simulink model "C_3_2020b"  (R2021a)
settings: Solver=VariableStepAuto  StartTime=0.0  StopTime=10.0  RelTol=1e-3
undefined symbols (not defined in the file or in its folder): pendubot_eqt, pendubot_reg, Ts
libraries: simulink x2
settings Model: Creator=afons  LastModifiedBy=Colin
settings SolverCC: AlgebraicLoopSolver=TrustRegion
settings DebuggingCC: UnconnectedInputMsg=none  UnconnectedOutputMsg=none  UnconnectedLineMsg=none  SFMachineParentedDataDiag=warning
settings ModelReferenceCC: EnableRefExpFcnMdlSchedulingChecks=off
settings RTWCC: Description=Generic Real-Time Target

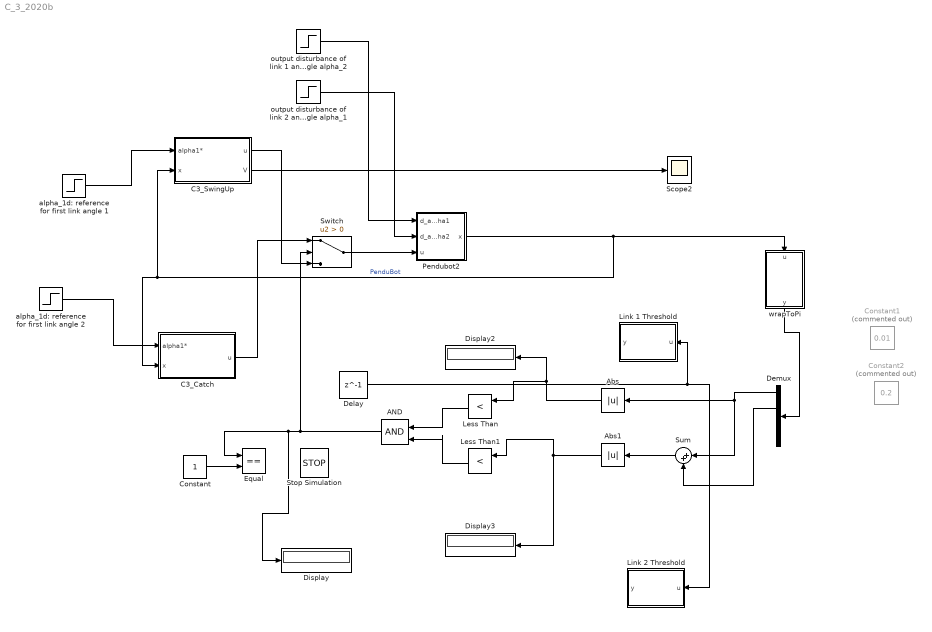
== system C_3_2020b ==
  AND : Logic  IconShape=distinctive  AllPortsSameDT=off  OutDataTypeStr=boolean
  Abs : Abs
  Abs1 : Abs
  C3_Catch : Subsystem
  C3_SwingUp : Subsystem
  Constant : Constant
  Constant1 : Constant  Commented=on  Value=0.01
  Constant2 : Constant  Commented=on  Value=0.2
  Delay : Delay  DelayLength=1
  Demux : Demux
  Display : Display
  Display2 : Display
  Display3 : Display
  Equal : RelationalOperator  Operator===  OutDataTypeStr=boolean  RndMeth=Simplest
  Less Than : RelationalOperator  Operator=<  OutDataTypeStr=boolean  RndMeth=Simplest
  Less Than1 : RelationalOperator  Operator=<  OutDataTypeStr=boolean  RndMeth=Simplest
  Link 1 Threshold : MATLAB Function  TreatAsAtomicUnit=on
  Link 2 Threshold : MATLAB Function  TreatAsAtomicUnit=on
  Pendubot2 : Subsystem  mask(Pendubot){x10=0, x20=0, x30=0, x40=0, Ts=Ts}
      mask prompts: x10 "Initial angle of link 1:"; x20 "Initial angular speed for link 1 :"; x30 "Initial angle of link 2 :"; x40 "Initial angular speed for link 2 :"; Ts "Sampling time [s] :"
      mask help: Initial conditions (initial state)
      mask Display:
      | plot(0.1*[1 9],0.1*[1 1])
      | plot(0.1*[1.5 1.5 8.5 8.5],0.1*[1 4 4 1])
      | plot(0.1*[5.2 8.2],0.1*[1 5])
      | plot(0.1*[4.8 7.8],0.1*[1 5])
      | plot(0.1*[7.8 5.8],0.1*[5 9.5])
      | plot(0.1*[8.2 6.2],0.1*[5 9.5])
  Scope2 : Scope
  Stop Simulation : Stop
  Sum : Sum  Inputs=|++
  Switch : Switch  Criteria=u2 > Threshold
  alpha_1d: reference for first link angle 1 : Step  Time=2  After=pi  SampleTime=Ts
  alpha_1d: reference for first link angle 2 : Step  Time=2  After=pi  SampleTime=Ts
  output disturbance of link 1 angle alpha_2 : Step  Time=5  After=0  SampleTime=Ts
  output disturbance of link 2 angle alpha_1 : Step  Time=2  After=0  SampleTime=Ts
  wrapToPi : MATLAB Function  TreatAsAtomicUnit=on
  wires:
  C3_SwingUp/2(V) -> Scope2/1
  output disturbance of link 2 angle alpha_1/1 -> Pendubot2/2(d_alpha2)
  Switch/1 -> Pendubot2/3(u)
  output disturbance of link 1 angle alpha_2/1 -> Pendubot2/1(d_alpha1)
  Pendubot2/1(x) -> C3_Catch/2(x), C3_SwingUp/2(x), wrapToPi/1(u)  "PenduBot"
  alpha_1d: reference for first link angle 1/1 -> C3_SwingUp/1(alpha1*)
  C3_SwingUp/1(u) -> Switch/3
  Constant/1 -> Equal/2
  C3_Catch/1(u) -> Switch/1
  alpha_1d: reference for first link angle 2/1 -> C3_Catch/1(alpha1*)
  Less Than/1 -> AND/1
  Demux/2 -> Sum/2
  Less Than1/1 -> AND/2
  Sum/1 -> Abs1/1
  wrapToPi/1(y) -> Demux/1
  Abs/1 -> Display2/1, Less Than/1
  Demux/1 -> Abs/1, Sum/1
  Abs1/1 -> Display3/1, Less Than1/1
  AND/1 -> Switch/2, Display/1, Equal/1
  Delay/1 -> Link 2 Threshold/1(u), Link 1 Threshold/1(u)

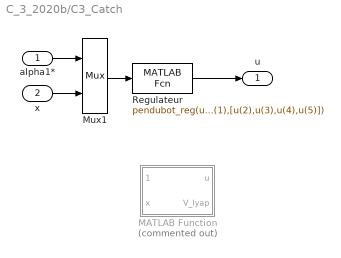
== system C_3_2020b/C3_Catch ==
  alpha1* : Inport
  x : Inport  Port=2
  MATLAB Function : MATLAB Function  Commented=on  TreatAsAtomicUnit=on
  Mux1 : Mux  Inputs=2
  Regulateur : MATLABFcn  MATLABFcn=pendubot_reg(u(1),[u(2),u(3),u(4),u(5)])
  u : Outport
  wires:
  Mux1/1 -> Regulateur/1
  alpha1*/1 -> Mux1/1
  x/1 -> Mux1/2
  Regulateur/1 -> u/1

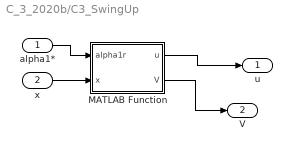
== system C_3_2020b/C3_SwingUp ==
  alpha1* : Inport
  x : Inport  Port=2
  MATLAB Function : MATLAB Function  TreatAsAtomicUnit=on
  u : Outport
  V : Outport  Port=2
  wires:
  alpha1*/1 -> MATLAB Function/1(alpha1r)
  x/1 -> MATLAB Function/2(x)
  MATLAB Function/1(u) -> u/1
  MATLAB Function/2(V) -> V/1

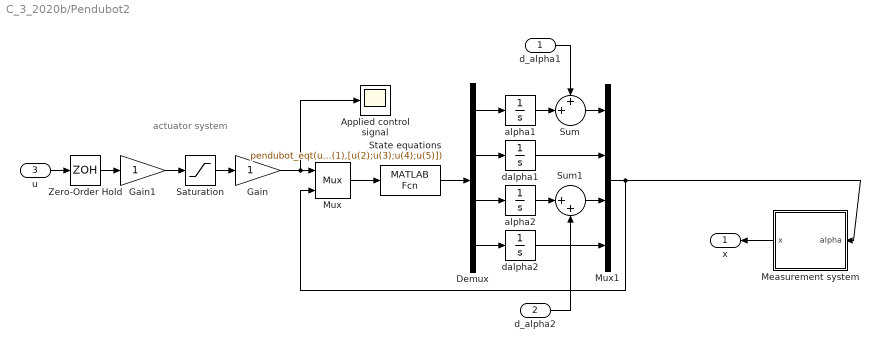
== system C_3_2020b/Pendubot2 ==
  note: actuator system
  d_alpha1 : Inport
  d_alpha2 : Inport  Port=2
  u : Inport  Port=3
  Applied control signal : Scope
  Demux : Demux
      settings: DisplayOption=none
  Gain : Gain  SaturateOnIntegerOverflow=on  OutDataTypeStr=Inherit: Same as input  ParamDataTypeStr=Inherit: Same as input
  Gain1 : Gain  SaturateOnIntegerOverflow=on  OutDataTypeStr=Inherit: Same as input  ParamDataTypeStr=Inherit: Same as input
  Measurement system : Subsystem
  Mux : Mux  Inputs=2
  Mux1 : Mux
  Saturation : Saturate  UpperLimit=10  LowerLimit=-10
  State equations : MATLABFcn  MATLABFcn=pendubot_eqt(u(1),[u(2);u(3);u(4);u(5)])  OutputDimensions=4
  Sum : Sum  Inputs=++|  InputSameDT=on  SaturateOnIntegerOverflow=on  OutDataTypeStr=Inherit: Same as first input
  Sum1 : Sum  Inputs=|++  InputSameDT=on  SaturateOnIntegerOverflow=on  OutDataTypeStr=Inherit: Same as first input
  Zero-Order Hold : ZeroOrderHold  SampleTime=Ts
  alpha1 : Integrator  InitialCondition=x10
  alpha2 : Integrator  InitialCondition=x30
  dalpha1 : Integrator  InitialCondition=x20
  dalpha2 : Integrator  InitialCondition=x40
  x : Outport
  wires:
  u/1 -> Zero-Order Hold/1
  State equations/1 -> Demux/1
  Mux/1 -> State equations/1
  Saturation/1 -> Gain/1
  Zero-Order Hold/1 -> Gain1/1
  Gain1/1 -> Saturation/1
  Gain/1 -> Mux/1, Applied control signal/1
  Mux1/1 -> Mux/2, Measurement system/1(alpha)
  dalpha2/1 -> Mux1/4
  Demux/1 -> alpha1/1
  Demux/2 -> dalpha1/1
  Demux/3 -> alpha2/1
  Demux/4 -> dalpha2/1
  Sum/1 -> Mux1/1
  Sum1/1 -> Mux1/3
  dalpha1/1 -> Mux1/2
  alpha1/1 -> Sum/2
  d_alpha1/1 -> Sum/1
  alpha2/1 -> Sum1/1
  d_alpha2/1 -> Sum1/2
  Measurement system/1(x) -> x/1

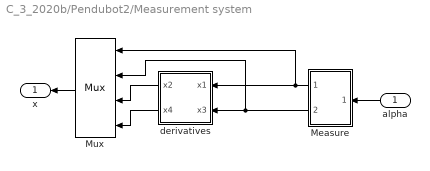
== system C_3_2020b/Pendubot2/Measurement system ==
  alpha : Inport
  Measure : Subsystem
  Mux : Mux
  derivatives : Subsystem
  x : Outport
  wires:
  derivatives/2(x4) -> Mux/4
  Mux/1 -> x/1
  Measure/1(xm(1)) -> derivatives/1(x1), Mux/1
  alpha/1 -> Measure/1(alpha)
  Measure/2(xm(1)1) -> derivatives/2(x3), Mux/2
  derivatives/1(x2) -> Mux/3

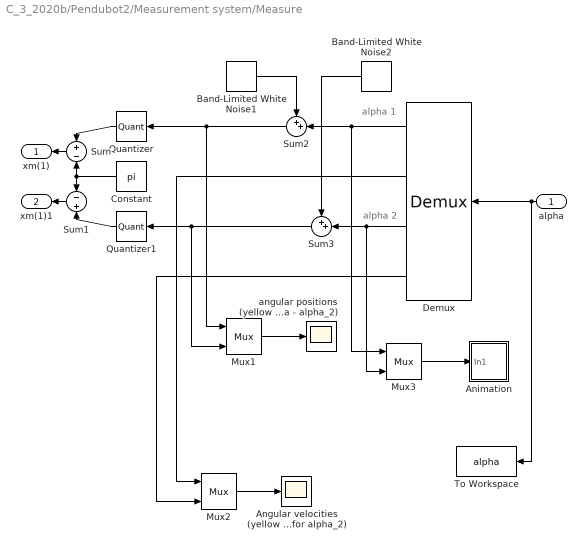
== system C_3_2020b/Pendubot2/Measurement system/Measure ==
  note: alpha 1
  note: alpha 2
  alpha : Inport
  "Angular velocities (yellow - for alpha_1, magenta - for alpha_2) " : Scope
  Animation : Subsystem  mask(Animation Block){ts=10*0.003}
      mask prompts: ts "Sample time:"
      mask Display: plot([.1,.9],[.9,.9],[.5,.2],[.9,.25],[.475,.475,.525,.525,.475],[.875,.925,.925,.875,.875])
  Band-Limited White Noise1 : simulink/Sources/Band-Limited White Noise  Cov=[1e-8]  Ts=Ts  seed=[23341]
  Band-Limited White Noise2 : simulink/Sources/Band-Limited White Noise  Cov=[1e-7]  Ts=Ts  seed=[32214]
  Constant : Constant  Value=pi
  Demux : Demux
      settings: DisplayOption=none
  Mux1 : Mux  Inputs=2
  Mux2 : Mux  Inputs=2
  Mux3 : Mux  Inputs=2
  Quantizer : Quantizer  QuantizationInterval=2*pi/5000
  Quantizer1 : Quantizer  QuantizationInterval=2*pi/5000
  Sum : Sum  Inputs=+-  InputSameDT=on  SaturateOnIntegerOverflow=on  OutDataTypeStr=Inherit: Same as first input
  Sum1 : Sum  Inputs=-+  InputSameDT=on  SaturateOnIntegerOverflow=on  OutDataTypeStr=Inherit: Same as first input
  Sum2 : Sum  Inputs=++|  InputSameDT=on  SaturateOnIntegerOverflow=on  OutDataTypeStr=Inherit: Same as first input
  Sum3 : Sum  Inputs=++|  InputSameDT=on  SaturateOnIntegerOverflow=on  OutDataTypeStr=Inherit: Same as first input
  To Workspace : ToWorkspace  VariableName=alpha  SampleTime=Ts
  "angular positions (yellow - alpha_1, magenta - alpha_2)" : Scope
  xm(1) : Outport  Tag=alpha1
  xm(1)1 : Outport  Port=2
  wires:
  alpha/1 -> To Workspace/1, Demux/1
  Demux/2 -> Mux2/1
  Demux/4 -> Mux2/2
  Mux2/1 -> "Angular velocities (yellow - for alpha_1, magenta - for alpha_2) "/1
  Sum/1 -> xm(1)/1
  Quantizer/1 -> Sum/1
  Sum1/1 -> xm(1)1/1
  Quantizer1/1 -> Sum1/2
  Constant/1 -> Sum/2, Sum1/1
  Band-Limited White Noise1/1 -> Sum2/1
  Band-Limited White Noise2/1 -> Sum3/1
  Sum2/1 -> Quantizer/1, Mux1/1
  Sum3/1 -> Quantizer1/1, Mux1/2
  Mux1/1 -> "angular positions (yellow - alpha_1, magenta - alpha_2)"/1
  Demux/1 -> Sum2/2, Mux3/1
  Demux/3 -> Sum3/2, Mux3/2
  Mux3/1 -> Animation/1(In1)

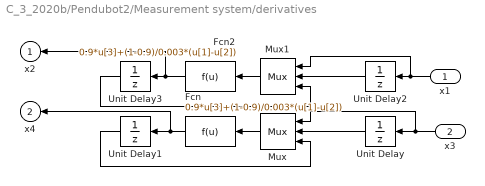
== system C_3_2020b/Pendubot2/Measurement system/derivatives ==
  x1 : Inport
  x3 : Inport  Port=2
  Fcn : Fcn  Expr=0.9*u[3]+(1-0.9)/0.003*(u[1]-u[2])
  Fcn2 : Fcn  Expr=0.9*u[3]+(1-0.9)/0.003*(u[1]-u[2])
  Mux : Mux  Inputs=3
  Mux1 : Mux  Inputs=3
  Unit Delay{,1..3} (4 alike) : UnitDelay  SampleTime=Ts  HasFrameUpgradeWarning=on
  x2 : Outport
  x4 : Outport  Port=2
  wires:
  Unit Delay/1 -> Mux/2
  Mux/1 -> Fcn/1
  Unit Delay1/1 -> Mux/3
  Fcn/1 -> Unit Delay1/1, x4/1
  x3/1 -> Unit Delay/1, Mux/1
  Unit Delay2/1 -> Mux1/2
  Mux1/1 -> Fcn2/1
  Unit Delay3/1 -> Mux1/3
  x1/1 -> Unit Delay2/1, Mux1/1
  Fcn2/1 -> Unit Delay3/1, x2/1

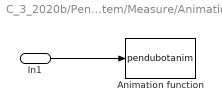
== system C_3_2020b/Pendubot2/Measurement system/Measure/Animation ==
  In1 : Inport
  Animation function : S-Function  FunctionName=pendubotanim  Parameters=ts  SFunctionDeploymentMode=off  EnableBusSupport=off
      settings: DeleteFcn=if ~isempty(findobj('type','figure','name','simppend Animation'));close('simppend Animation'); end;
  wires:
  In1/1 -> Animation function/1

== matlab function C_3_2020b/wrapToPi ==
  data: u input; y output
function y = fcn(u)

y = wrapToPi(u);

== matlab function C_3_2020b/C3_Catch/MATLAB Function ==
  data: alpha1r input; u output; x input; V_lyap output
function [u, V_lyap] = pendulumNonLinear(alpha1r,x)
%UNTITLED Summary of this function goes here
%   Detailed explanation goes here
    alpha1 = x(1);
    alpha2 = x(2);
    dalpha1 = x(3);
    dalpha2 = x(4);

    p1 = 0.0148; p2 = 0.0051; p3 = 0.0046; p4 = 0.1003; p5 = 0.0303;
    g = 9.81;
    E_ref = (p4 + p5) * g;

    % Mass matrix M(alpha)
    M = [p1 + p2 + 2*p3*cos(alpha2 - alpha1), p2 + p3*cos(alpha2 - alpha1);
         p2 + p3*cos(alpha2 - alpha1), p2];

    % Potential energy V
    V = -p4*g*cos(alpha1) - p5*g*cos(alpha2);

    % Kinetic energy T
    T = 0.5 * [dalpha1 dalpha2] * M * [dalpha1; dalpha2];

    % Total energy
    E = T + V;

    % Lyapunov Function (Energy-based)
    V_lyap = E;
    k_p = 0.5;
    k_d = 0.1;
    % Derivative of the Lyapunov Function
    dV_lyap = [dalpha1; dalpha2]' * (0.5 * M * [dalpha1; dalpha2] + [p4*g*sin(alpha1); p5*g*sin(alpha2)]);

    corr_x = [x(1) ; x(2) ; x(3) ; x(4)];
    % Control Law for Swing-Up using PD controller
    u = -k_p * corr_x;

end

== matlab function C_3_2020b/Link 1 Threshold ==
  data: u input; y output
function y = fcn(u)
if u == 1
    y = 100;
else
    y = 0.01;
end

== matlab function C_3_2020b/Link 2 Threshold ==
  data: u input; y output
function y = fcn(u)
if u == 1
    y = 200;
else
    y = 0.2;
end

== matlab function C_3_2020b/C3_SwingUp/MATLAB Function ==
  data: alpha1r input; u output; x input; V output
function [u, V] = pendubot_C3(alpha1r,x)

a1 = x(1);
a2 = x(2);
da1 = x(3);
da2 = x(4);

% Define Constants
p1 = 0.0148;
p2 = 0.0051;
p3 = 0.0046;
p4 = 0.1003;
p5 = 0.0303;
grav  = 9.81;
torque = 3.9621;
k = 3.9621/8;
% tau = [torque ; 0];

% Dynamic Matrices

M  = [p1+p2+p3*cos(a2), p2+p3*cos(a2); p2+p3*cos(a2), p2];
C = p3*sin(a2) * [-da2 , -da1 - da2 ; -da1 , 0];
G  = [p4*grav*cos(a1) + p5 * grav * cos(a1 + a2); p5*grav*cos(a2 + a1)];
F = [0.00545 * da1 + 0.0023 * tanh(30 * da1) ; 0.00047 * da2 + 0.0025 * tanh(30 * da2)];

% Energy Data

U = p4 * sin(a1) + p5 * sin(a1 + a2);

K = 0.5 * [da1 , da2] * M * [da1 ; da2];
% dK = [da1 , da2] * (tau - C * [da1 ; da2] - G - F) + 0.5 * [da1 , da2] * dM * [da1 ; da2];

E = K + U;

E_TOP = (p4 + p5) * grav;

E_est = E - E_TOP;

% Lyapunov Data

kk = 0.1;  %6.359;
kd = 30; %8.71;
a1_est = a1 - alpha1r;
a2_est = a1 + a2 - alpha1r;

V = kk * K + 0.5 * [a1_est , a2_est] * kd * [a1_est ; a2_est];

% Control Law
G_1 = p4 * grav * sin(a1);
tau = -1/kk * (da1 + kd * a1_est) + G_1 ;
u = tau;
end
